simulink model "sim_qn5"  (R2022b)
settings: Solver=ode4  StartTime=0.0  StopTime=10.0  FixedStep=tstep  RelTol=1e-3
undefined symbols (not defined in the file): den, num
libraries: simulink x1
settings Model: Creator=dipte  LastModifiedBy=dipte
settings DataIOCC: ReturnWorkspaceOutputs=off

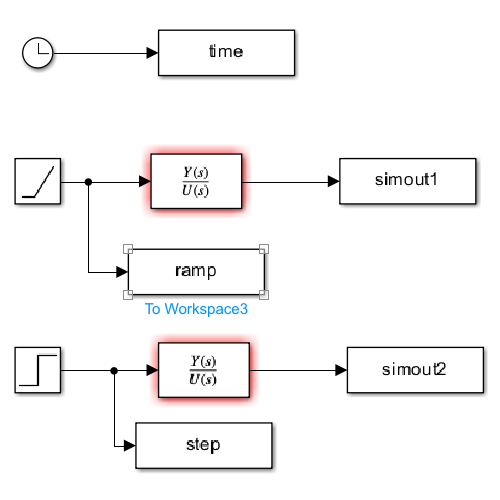
[thumbnail: Simulink's stored preview of the top-level diagram]
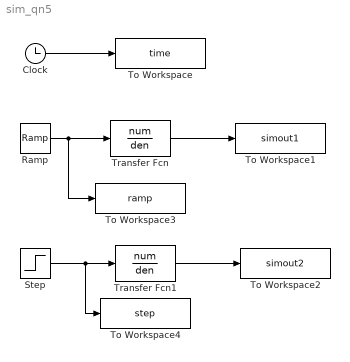
== system sim_qn5 ==
  Clock : Clock
  Ramp : simulink/Sources/Ramp  slope=1  start=0  InitialOutput=0
  Step : Step  Time=0  SampleTime=0
  To Workspace : ToWorkspace  VariableName=time  SampleTime=-1
      settings: Save2DSignal=2-D array (concatenate along first dimension)
  To Workspace1 : ToWorkspace  VariableName=simout1  SampleTime=-1
      settings: Save2DSignal=2-D array (concatenate along first dimension)
  To Workspace2 : ToWorkspace  VariableName=simout2  SampleTime=-1
      settings: Save2DSignal=2-D array (concatenate along first dimension)
  To Workspace3 : ToWorkspace  VariableName=ramp  SampleTime=-1
      settings: Save2DSignal=2-D array (concatenate along first dimension)
  To Workspace4 : ToWorkspace  VariableName=step  SampleTime=-1
      settings: Save2DSignal=2-D array (concatenate along first dimension)
  Transfer Fcn : TransferFcn  Numerator=num  Denominator=den
  Transfer Fcn1 : TransferFcn  Numerator=num  Denominator=den
  wires:
  Step/1 -> To Workspace4/1, Transfer Fcn1/1
  Transfer Fcn1/1 -> To Workspace2/1
  Ramp/1 -> To Workspace3/1, Transfer Fcn/1
  Transfer Fcn/1 -> To Workspace1/1
  Clock/1 -> To Workspace/1
